simulink model "Waveforms"  (R2021b)
settings: Solver=VariableStepAuto  StartTime=0.0  StopTime=300  RelTol=1e-3
undefined symbols (not defined in the file or in its folder): Ts
libraries: simulink x10
settings Model: Creator=danif  LastModifiedBy=danif

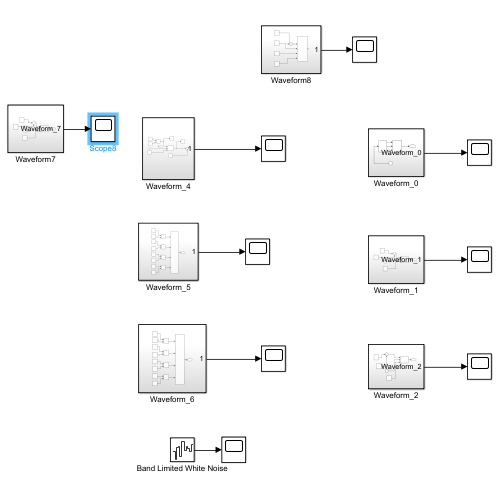
[thumbnail: Simulink's stored preview of the top-level diagram]
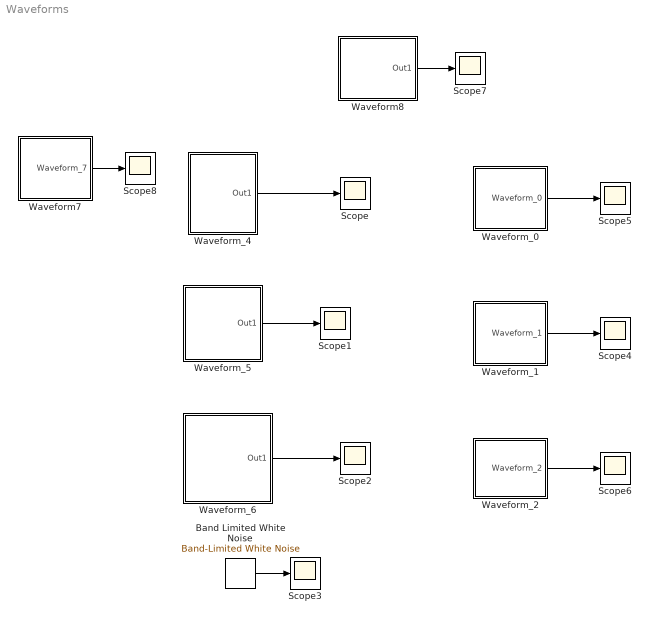
== system Waveforms ==
  Band Limited White Noise : simulink/Sources/Band-Limited White Noise  Cov=[0.01]  Ts=0.1  seed=[23341]
  Scope{,1..8} (9 alike) : Scope
  Waveform7 : Subsystem
  Waveform8 : Subsystem
  Waveform_0 : Subsystem
  Waveform_1 : Subsystem
  Waveform_2 : Subsystem
  Waveform_4 : Subsystem
  Waveform_5 : Subsystem
  Waveform_6 : Subsystem
  wires:
  Waveform_4/1(Out1) -> Scope/1
  Waveform_6/1(Out1) -> Scope2/1
  Waveform_5/1(Out1) -> Scope1/1
  Band Limited White Noise/1 -> Scope3/1
  Waveform_1/1(Waveform_1) -> Scope4/1
  Waveform_0/1(Waveform_0) -> Scope5/1
  Waveform_2/1(Waveform_2) -> Scope6/1
  Waveform8/1(Out1) -> Scope7/1
  Waveform7/1(Waveform_7) -> Scope8/1

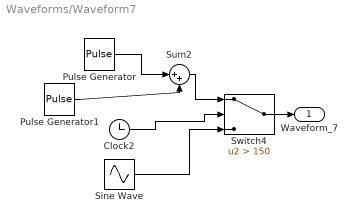
== system Waveforms/Waveform7 ==
  Clock2 : Clock
  Pulse Generator : DiscretePulseGenerator  PulseType=Time based  Amplitude=0.6  Period=120  PulseWidth=15
  Pulse Generator1 : DiscretePulseGenerator  PulseType=Time based  Amplitude=-0.6  Period=120  PulseWidth=15  PhaseDelay=60
  Sine Wave : Sin  Amplitude=0.6  Frequency=0.2  SampleTime=Ts
  Sum2 : Sum  Inputs=|++
  Switch4 : Switch  Criteria=u2 > Threshold  Threshold=150
  Waveform_7 : Outport
  wires:
  Clock2/1 -> Switch4/2
  Sum2/1 -> Switch4/1
  Pulse Generator1/1 -> Sum2/2
  Pulse Generator/1 -> Sum2/1
  Sine Wave/1 -> Switch4/3
  Switch4/1 -> Waveform_7/1

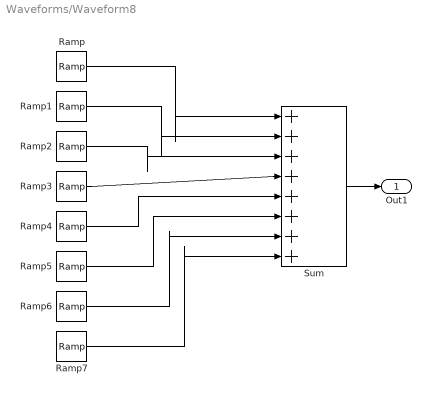
== system Waveforms/Waveform8 ==
  Ramp : simulink/Sources/Ramp  slope=0.005  start=50  InitialOutput=0
  Ramp1 : simulink/Sources/Ramp  slope=-0.005  start=75  InitialOutput=0
  Ramp2 : simulink/Sources/Ramp  slope=-0.005  start=100  InitialOutput=0
  Ramp3 : simulink/Sources/Ramp  slope=0.005  start=125  InitialOutput=0
  Ramp4 : simulink/Sources/Ramp  slope=-0.005  start=150  InitialOutput=0
  Ramp5 : simulink/Sources/Ramp  slope=+0.005  start=175  InitialOutput=0
  Ramp6 : simulink/Sources/Ramp  slope=0.005  start=195  InitialOutput=0
  Ramp7 : simulink/Sources/Ramp  slope=-0.005  start=220  InitialOutput=0
  Sum : Sum  Inputs=|++++++++
  Out1 : Outport
  wires:
  Ramp2/1 -> Sum/3
  Ramp1/1 -> Sum/2
  Ramp3/1 -> Sum/4
  Ramp/1 -> Sum/1
  Sum/1 -> Out1/1
  Ramp7/1 -> Sum/8
  Ramp6/1 -> Sum/7
  Ramp5/1 -> Sum/6
  Ramp4/1 -> Sum/5

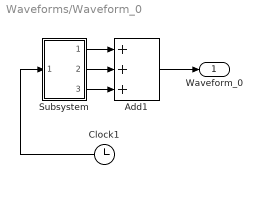
== system Waveforms/Waveform_0 ==
  Add1 : Sum  Inputs=+++
  Clock1 : Clock
  Subsystem : Subsystem
  Waveform_0 : Outport
  wires:
  Clock1/1 -> Subsystem/1(In1)
  Subsystem/2(Out2) -> Add1/2
  Subsystem/1(Out1) -> Add1/1
  Subsystem/3(Out3) -> Add1/3
  Add1/1 -> Waveform_0/1

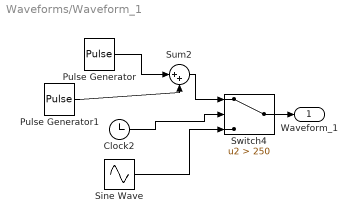
== system Waveforms/Waveform_1 ==
  Clock2 : Clock
  Pulse Generator : DiscretePulseGenerator  PulseType=Time based  Amplitude=0.6  Period=120  PulseWidth=15
  Pulse Generator1 : DiscretePulseGenerator  PulseType=Time based  Amplitude=-0.6  Period=120  PulseWidth=15  PhaseDelay=60
  Sine Wave : Sin  Amplitude=0.6  Frequency=0.2  SampleTime=Ts
  Sum2 : Sum  Inputs=|++
  Switch4 : Switch  Criteria=u2 > Threshold  Threshold=250
  Waveform_1 : Outport
  wires:
  Clock2/1 -> Switch4/2
  Sum2/1 -> Switch4/1
  Pulse Generator1/1 -> Sum2/2
  Pulse Generator/1 -> Sum2/1
  Sine Wave/1 -> Switch4/3
  Switch4/1 -> Waveform_1/1

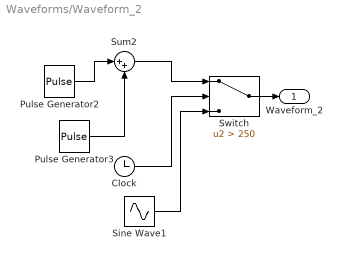
== system Waveforms/Waveform_2 ==
  Clock : Clock
  Pulse Generator2 : DiscretePulseGenerator  PulseType=Time based  Amplitude=0.2  Period=120  PulseWidth=50
  Pulse Generator3 : DiscretePulseGenerator  PulseType=Time based  Amplitude=-0.2  Period=120  PulseWidth=50  PhaseDelay=60
  Sine Wave1 : Sin  Amplitude=0.2  Frequency=0.2  SampleTime=Ts
  Sum2 : Sum  Inputs=|++
  Switch : Switch  Criteria=u2 > Threshold  Threshold=250
  Waveform_2 : Outport
  wires:
  Pulse Generator2/1 -> Sum2/1
  Sine Wave1/1 -> Switch/3
  Clock/1 -> Switch/2
  Pulse Generator3/1 -> Sum2/2
  Sum2/1 -> Switch/1
  Switch/1 -> Waveform_2/1

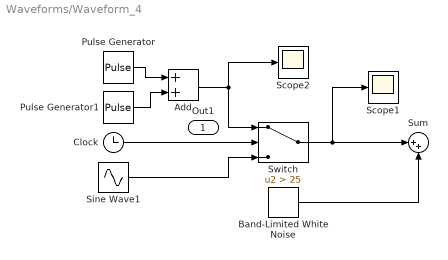
== system Waveforms/Waveform_4 ==
  Add : Sum
  Band-Limited White Noise : simulink/Sources/Band-Limited White Noise  Cov=[0.0001]  Ts=0.1  seed=[23341]
  Clock : Clock
  Pulse Generator : DiscretePulseGenerator  PulseType=Time based  Amplitude=0.3  Period=30  PulseWidth=25
  Pulse Generator1 : DiscretePulseGenerator  PulseType=Time based  Amplitude=-0.5  Period=30  PulseWidth=25  PhaseDelay=15
  Scope1 : Scope
  Scope2 : Scope
  Sine Wave1 : Sin  Amplitude=0.3  Frequency=0.2  SampleTime=0.1
  Sum : Sum  Inputs=|++
  Switch : Switch  Criteria=u2 > Threshold  Threshold=25
  Out1 : Outport
  wires:
  Clock/1 -> Switch/2
  Sine Wave1/1 -> Switch/3
  Add/1 -> Scope2/1, Switch/1
  Switch/1 -> Sum/1, Scope1/1
  Pulse Generator/1 -> Add/1
  Band-Limited White Noise/1 -> Sum/2
  Pulse Generator1/1 -> Add/2

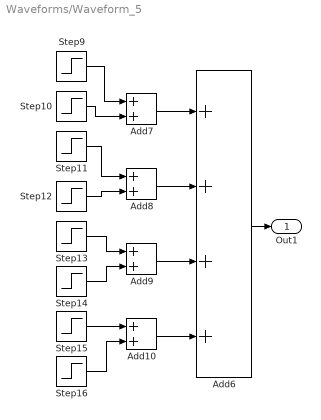
== system Waveforms/Waveform_5 ==
  Add{7..10} (4 alike) : Sum
  Add6 : Sum  Inputs=++++
  Step10 : Step  Time=45  After=-0.46  SampleTime=Ts
  Step11 : Step  Time=105  After=-0.46  SampleTime=Ts
  Step12 : Step  Time=125  After=0.46  SampleTime=Ts
  Step13 : Step  Time=185  After=0.5  SampleTime=Ts
  Step14 : Step  Time=195  After=-0.5  SampleTime=0
  Step15 : Step  Time=230  After=-0.5  SampleTime=Ts
  Step16 : Step  Time=240  After=0.5  SampleTime=Ts
  Step9 : Step  Time=30  After=0.46  SampleTime=Ts
  Out1 : Outport
  wires:
  Add7/1 -> Add6/1
  Step9/1 -> Add7/1
  Step13/1 -> Add9/1
  Step14/1 -> Add9/2
  Step12/1 -> Add8/2
  Add10/1 -> Add6/4
  Step16/1 -> Add10/2
  Step10/1 -> Add7/2
  Add9/1 -> Add6/3
  Add8/1 -> Add6/2
  Step15/1 -> Add10/1
  Step11/1 -> Add8/1
  Add6/1 -> Out1/1

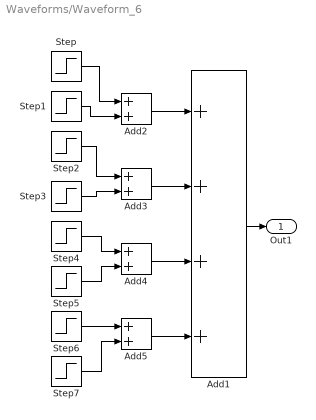
== system Waveforms/Waveform_6 ==
  Add1 : Sum  Inputs=++++
  Add{2..5} (4 alike) : Sum
  Step : Step  Time=20  After=-0.5  SampleTime=0
  Step1 : Step  Time=30  After=0.5  SampleTime=0
  Step2 : Step  Time=90  After=-0.33  SampleTime=0
  Step3 : Step  Time=105  After=0.33  SampleTime=0
  Step4 : Step  Time=155  After=0.5  SampleTime=0
  Step5 : Step  Time=175  After=-0.5  SampleTime=0
  Step6 : Step  Time=235  After=0.6  SampleTime=0
  Step7 : Step  Time=245  After=-0.6  SampleTime=0
  Out1 : Outport
  wires:
  Add5/1 -> Add1/4
  Add4/1 -> Add1/3
  Step4/1 -> Add4/1
  Step/1 -> Add2/1
  Step2/1 -> Add3/1
  Step5/1 -> Add4/2
  Add3/1 -> Add1/2
  Step7/1 -> Add5/2
  Step1/1 -> Add2/2
  Step6/1 -> Add5/1
  Step3/1 -> Add3/2
  Add2/1 -> Add1/1
  Add1/1 -> Out1/1

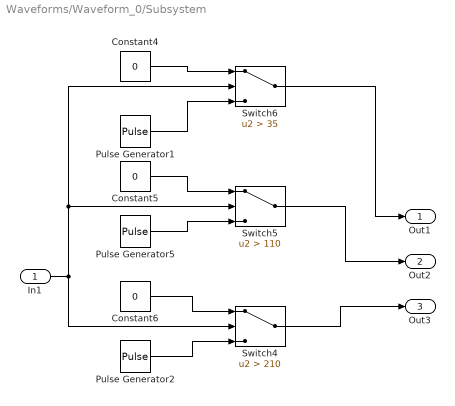
== system Waveforms/Waveform_0/Subsystem ==
  In1 : Inport
  Constant4 : Constant  Value=0
  Constant5 : Constant  Value=0
  Constant6 : Constant  Value=0
  Pulse Generator1 : DiscretePulseGenerator  PulseType=Time based  Amplitude=0.7  Period=30  PulseWidth=50  PhaseDelay=20
  Pulse Generator2 : DiscretePulseGenerator  PulseType=Time based  Amplitude=-0.27  Period=40  PulseWidth=50  PhaseDelay=190
  Pulse Generator5 : DiscretePulseGenerator  PulseType=Time based  Amplitude=-0.4  Period=30  PulseWidth=50  PhaseDelay=95
  Switch4 : Switch  Criteria=u2 > Threshold  Threshold=210
  Switch5 : Switch  Criteria=u2 > Threshold  Threshold=110
  Switch6 : Switch  Criteria=u2 > Threshold  Threshold=35
  Out1 : Outport
  Out2 : Outport  Port=2
  Out3 : Outport  Port=3
  wires:
  In1/1 -> Switch4/2, Switch5/2, Switch6/2
  Pulse Generator1/1 -> Switch6/3
  Constant5/1 -> Switch5/1
  Constant6/1 -> Switch4/1
  Switch4/1 -> Out3/1
  Pulse Generator5/1 -> Switch5/3
  Switch6/1 -> Out1/1
  Constant4/1 -> Switch6/1
  Pulse Generator2/1 -> Switch4/3
  Switch5/1 -> Out2/1
